simulink model "s5_3"  (Simulink 6.6)
settings: Solver=ode45  SolverMode=SingleTasking  StartTime=0.0  StopTime=t_d  FixedStep=Tc  MaxStep=Tc  RelTol=1e-8  AbsTol=1e-8
values from neighbouring files (symbols this model uses):
  F_m = 0.01    [i5_3.m]
  G_v = 1    [i5_3.m]
  I_m = 0.0014    [i5_3.m]
  k_i = 1    [i5_3.m]
  K_i = 21592    [i5_3.m]
  k_t = 0.2    [i5_3.m]
  k_v = 0.2    [i5_3.m]
  L_a = 2e-3    (= 0.002)    [i5_3.m]
  R_a = 0.2    [i5_3.m]
  T_i = 9/21592    (= 0.000416821044831)    [i5_3.m]
  T_v = 0.1e-3    (= 0.0001)    [i5_3.m]
  Ts = Tc    (= 0.0001)    [i5_3.m]
settings Model: Creator=luigivillani  LastModifiedBy=luigivillani  ExtModeAutoUpdateStatusClock=off
settings SolverCC: InitialStep=0.1*Tc
settings DataIOCC: LimitDataPoints=off  SaveOutput=off  SaveTime=off
settings OptimizationCC: BlockReduction=off  BooleanDataType=off
settings DebuggingCC: SignalResolutionControl=TryResolveAllWithWarning  SolverPrmCheckMsg=none  MultiTaskDSMMsg=warning  MultiTaskCondExecSysMsg=none  StrictBusMsg=None
settings HardwareCC: TargetUnknown=on
settings RTWCC: IncludeERTFirstTime=on

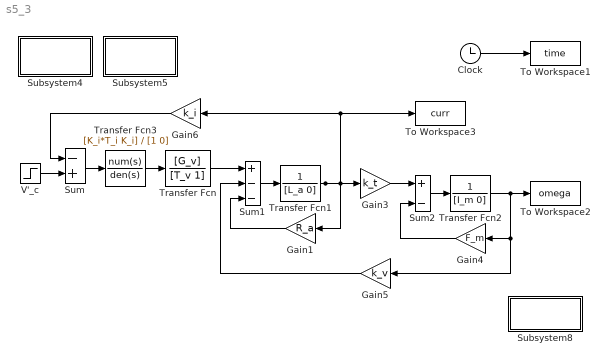
== system s5_3 ==
  Clock : Clock
  Gain1 : Gain  Orientation=left  Gain=R_a  SaturateOnIntegerOverflow=on
      mask Display: disp('R_a')
  Gain3 : Gain  Gain=k_t  SaturateOnIntegerOverflow=on
      mask Display: disp('k_t')
  Gain4 : Gain  Orientation=left  Gain=F_m  SaturateOnIntegerOverflow=on
      mask Display: disp('F_m')
  Gain5 : Gain  Orientation=left  Gain=k_v  SaturateOnIntegerOverflow=on
      mask Display: disp('k_v')
  Gain6 : Gain  Orientation=left  Gain=k_i  SaturateOnIntegerOverflow=on
      mask Display: disp('k_i')
  Subsystem4 : Subsystem
      settings: OpenFcn=clear all;c=0;i5_3;
      mask Display: disp('current')
  Subsystem5 : Subsystem
      settings: OpenFcn=clear all;c=1;i5_3;
      mask Display: disp('velocity')
  Subsystem8 : Subsystem  Orientation=left
      settings: OpenFcn=p5_3;
      mask Display: disp('plot')
  Sum : Sum  Inputs=-+  SaturateOnIntegerOverflow=on  InputSameDT=on
  Sum1 : Sum  Inputs=+--  SaturateOnIntegerOverflow=on  InputSameDT=on
  Sum2 : Sum  Inputs=+-  SaturateOnIntegerOverflow=on  InputSameDT=on
  To Workspace1 : ToWorkspace  VariableName=time  SampleTime=Ts  SaveFormat=Array
      settings: MaxDataPoints=50001
  To Workspace2 : ToWorkspace  VariableName=omega  SampleTime=Ts  SaveFormat=Array
      settings: MaxDataPoints=50001
  To Workspace3 : ToWorkspace  VariableName=curr  SampleTime=Ts  SaveFormat=Array
      settings: MaxDataPoints=50001
  Transfer Fcn : TransferFcn  Numerator=[G_v]  Denominator=[T_v 1]
  Transfer Fcn1 : TransferFcn  Denominator=[L_a 0]
  Transfer Fcn2 : TransferFcn  Denominator=[I_m 0]
  Transfer Fcn3 : TransferFcn  Numerator=[K_i*T_i K_i]  Denominator=[1 0]
      mask Display: disp('C_i(s)')
  V'_c : Step  Time=0.0001  SampleTime=0
  wires:
  V'_c/1 -> Sum/2
  Sum/1 -> Transfer Fcn3/1
  Transfer Fcn/1 -> Sum1/1
  Sum1/1 -> Transfer Fcn1/1
  Gain3/1 -> Sum2/1
  Sum2/1 -> Transfer Fcn2/1
  Gain4/1 -> Sum2/2
  Transfer Fcn1/1 -> Gain3/1, Gain1/1, Gain6/1, To Workspace3/1
  Gain1/1 -> Sum1/3
  Gain5/1 -> Sum1/2
  Gain6/1 -> Sum/1
  Clock/1 -> To Workspace1/1
  Transfer Fcn3/1 -> Transfer Fcn/1
  Transfer Fcn2/1 -> Gain5/1, Gain4/1, To Workspace2/1

== system s5_3/Subsystem4 ==
  note: start

== system s5_3/Subsystem5 ==
  note: start

== system s5_3/Subsystem8 ==
  note: start
